simulink library "LIB_TF_G_12_StepControl"  (Simulink 8.6)
settings: Solver=ode45  StartTime=0.0  StopTime=10.0  RelTol=1e-3
PreLoadFcn:
  | if exist('tl_preloadfcn','file'), tl_preloadfcn(gcs,402); end
PostLoadFcn:
  | if exist('tl_postloadfcn','file'), tl_postloadfcn(gcs,402); end
undefined symbols (not defined in the file): ddv, u2, u3
libraries: tllib x4, LIB_TF_G_12_StepControl x1
(part 4 of 7)

== system LIB_TF_G_12_StepControl/TF_G_12_ControlStepExecution/New Step started/Adapt Step Target Value/Temperature Weighted ==
  s8_StepOrderValue : Inport
  u16_Temperature : Inport  Port=2
  e_TemperatureCompensationType : Inport  Port=3
  Action Port : ActionPort
  Data Type Conversion : DataTypeConversion
  If : If  NumInputs=2  IfExpression=u1  ElseIfExpressions=u2
  Merge : Merge  Inputs=3  InitialOutput=64  mask(TL_Merge){data={'date',735951.66799226857}}
      settings: CopyFcn=if exist('tl_reset_reviewflag','file')==2,tl_reset_reviewflag(gcbh);end  DeleteFcn=if exist('delete_tlblock','file')==2,delete_tlblock(gcbh);end  NameChangeFcn=if exist('rename_tlblock','file')==2,rename_tlblock(gcbh);end  OpenFcn=if exist('tl_open_blockdlg','file')==2,tl_open_blockdlg(gcbh);else,open_system(gcbh,'parameter');end
      mask Help: eval(['if exist(''tl_online_help'',''file'') == 2, tl_online_help(''Topic'',''TL_Merge''),else, web([''jar:file:///'',matlabroot,''/help/toolbox/simulink/help.jar!/slref/' lower(get_param(gcbh,'Blocktype')) '.html''], ''-helpbrowser''),end'])
      mask Display: plot([-0.05, 1.05, NaN, -0.05, 1.05],[.01, .01, NaN, .99, .99])
  Relational Operator1 : RelationalOperator  Operator===  OutDataTypeStr=boolean  mask(TL_RelationalOperator){data={'date',735951.66799189814}}
      settings: DeleteFcn=if exist('delete_tlblock','file')==2,delete_tlblock(gcbh);end  NameChangeFcn=if exist('rename_tlblock','file')==2,rename_tlblock(gcbh);end  OpenFcn=if exist('tl_open_blockdlg','file')==2,tl_open_blockdlg(gcbh);else,open_system(gcbh,'parameter');end
      mask Help: eval(['if exist(''tl_online_help'',''file'') == 2, tl_online_help(''Topic'',''TL_RelationalOperator''),else, web([''jar:file:///'',matlabroot,''/help/toolbox/simulink/help.jar!/slref/' lower(get_param(gcbh,'Blocktype')) '.html''], ''-helpbrowser''),end'])
      mask Display: plot([-0.05, 1.05, NaN, -0.05, 1.05],[.01, .01, NaN, .99, .99])
  Relational Operator2 : RelationalOperator  Operator=>  OutDataTypeStr=boolean  mask(TL_RelationalOperator){data={'date',735951.66799165506}}
      settings: DeleteFcn=if exist('delete_tlblock','file')==2,delete_tlblock(gcbh);end  NameChangeFcn=if exist('rename_tlblock','file')==2,rename_tlblock(gcbh);end  OpenFcn=if exist('tl_open_blockdlg','file')==2,tl_open_blockdlg(gcbh);else,open_system(gcbh,'parameter');end
      mask Help: eval(['if exist(''tl_online_help'',''file'') == 2, tl_online_help(''Topic'',''TL_RelationalOperator''),else, web([''jar:file:///'',matlabroot,''/help/toolbox/simulink/help.jar!/slref/' lower(get_param(gcbh,'Blocktype')) '.html''], ''-helpbrowser''),end'])
      mask Display: plot([-0.05, 1.05, NaN, -0.05, 1.05],[.01, .01, NaN, .99, .99])
  Step Order Negative : Subsystem  TreatAsAtomicUnit=on
  Step Order Positive : Subsystem  TreatAsAtomicUnit=on
  Step Order equal 0 : Subsystem  TreatAsAtomicUnit=on
  Zero : Constant  Value=ddv('Common/KS8_ZERO')  mask(TL_Constant){data={'output',{'variable','Common/KS8_ZERO'},'date',735951.66798423615}}
      settings: CopyFcn=if exist('tl_reset_reviewflag','file')==2,tl_reset_reviewflag(gcbh);end  DeleteFcn=if exist('delete_tlblock','file')==2,delete_tlblock(gcbh);end  NameChangeFcn=if exist('rename_tlblock','file')==2,rename_tlblock(gcbh);end  OpenFcn=if exist('tl_open_blockdlg','file')==2,tl_open_blockdlg(gcbh);else,open_system(gcbh,'parameter');end
      mask Help: eval(['if exist(''tl_online_help'',''file'') == 2, tl_online_help(''Topic'',''TL_Constant''),else, web([''jar:file:///'',matlabroot,''/help/toolbox/simulink/help.jar!/slref/' lower(get_param(gcbh,'Blocktype')) '.html''], ''-helpbrowser''),end'])
      mask Display: plot([-0.05, 1.05, NaN, -0.05, 1.05],[.01, .01, NaN, .99, .99])
  Out1 : Outport  InitialOutput=64
  wires:
  s8_StepOrderValue/1 -> Relational Operator1/2, Relational Operator2/2
  Zero/1 -> Relational Operator1/1, Relational Operator2/1
  If/1 -> Step Order equal 0/Action
  Relational Operator1/1 -> If/1
  Relational Operator2/1 -> If/2
  If/2 -> Step Order Negative/Action
  If/3 -> Step Order Positive/Action
  u16_Temperature/1 -> Step Order Positive/1(u16_Temperature), Step Order Negative/1(u16_Temperature)
  e_TemperatureCompensationType/1 -> Step Order Positive/2(e_TemperatureCompensationType)
  Step Order equal 0/1(Out1) -> Merge/1
  Step Order Negative/1(Out1) -> Merge/2
  Step Order Positive/1(Out1) -> Merge/3
  Merge/1 -> Data Type Conversion/1
  Data Type Conversion/1 -> Out1/1

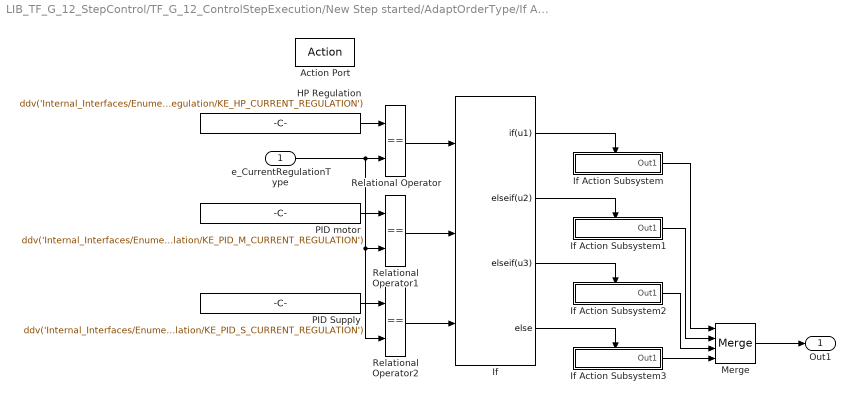
== system LIB_TF_G_12_StepControl/TF_G_12_ControlStepExecution/New Step started/AdaptOrderType/If Action Subsystem ==
  e_CurrentRegulationType : Inport  RequirementInfo={} %GIDa_189e736f_cca1_461e_9619_1829fc2b845e
  Action Port : ActionPort  RequirementInfo={} %GIDa_9c1052a9_2410_4f18_8ef4_d58b860af1af
  HP Regulation : Constant  Value=ddv('Internal_Interfaces/Enumerated_values/Current_Regulation/KE_HP_CURRENT_REGULATION')  mask(TL_Constant){data={'output',{'variable','Internal_Interfaces/Enumerated_values/Current_Regulation/KE_HP_CURRENT_REGULATION'},'date',735951.66798386571}}
      settings: CopyFcn=if exist('tl_reset_reviewflag','file')==2,tl_reset_reviewflag(gcbh);end  DeleteFcn=if exist('delete_tlblock','file')==2,delete_tlblock(gcbh);end  NameChangeFcn=if exist('rename_tlblock','file')==2,rename_tlblock(gcbh);end  OpenFcn=if exist('tl_open_blockdlg','file')==2,tl_open_blockdlg(gcbh);else,open_system(gcbh,'parameter');end
      mask Help: eval(['if exist(''tl_online_help'',''file'') == 2, tl_online_help(''Topic'',''TL_Constant''),else, web([''jar:file:///'',matlabroot,''/help/toolbox/simulink/help.jar!/slref/' lower(get_param(gcbh,'Blocktype')) '.html''], ''-helpbrowser''),end'])
      mask Display: plot([-0.05, 1.05, NaN, -0.05, 1.05],[.01, .01, NaN, .99, .99])
  If : If  RequirementInfo={} %GIDa_8698efec_5c77_4842_b73b_0b3a19be4617  NumInputs=3  IfExpression=u1  ElseIfExpressions=u2,u3
  If Action Subsystem : Subsystem  RequirementInfo={} %GIDa_4ad190b8_12b8_4004_92fb_b3b0c27a36d8  TreatAsAtomicUnit=on
  If Action Subsystem1 : Subsystem  RequirementInfo={} %GIDa_60d8e542_8624_44e2_88e0_16765795048d  TreatAsAtomicUnit=on
  If Action Subsystem2 : Subsystem  RequirementInfo={} %GIDa_c7e553bf_bc73_4930_9906_7d39347ac718  TreatAsAtomicUnit=on
  If Action Subsystem3 : Subsystem  RequirementInfo={} %GIDa_f2cbc51b_f895_475d_9a25_d84b280220b8  TreatAsAtomicUnit=on
  Merge : Merge  RequirementInfo={} %GIDa_b496a0a7_f35d_4795_a756_d7e1fdb3ad5a  Inputs=4  mask(TL_Merge){data={'date',735951.66797821759}}
      settings: CopyFcn=if exist('tl_reset_reviewflag','file')==2,tl_reset_reviewflag(gcbh);end  DeleteFcn=if exist('delete_tlblock','file')==2,delete_tlblock(gcbh);end  NameChangeFcn=if exist('rename_tlblock','file')==2,rename_tlblock(gcbh);end  OpenFcn=if exist('tl_open_blockdlg','file')==2,tl_open_blockdlg(gcbh);else,open_system(gcbh,'parameter');end
      mask Help: eval(['if exist(''tl_online_help'',''file'') == 2, tl_online_help(''Topic'',''TL_Merge''),else, web([''jar:file:///'',matlabroot,''/help/toolbox/simulink/help.jar!/slref/' lower(get_param(gcbh,'Blocktype')) '.html''], ''-helpbrowser''),end'])
      mask Display: plot([-0.05, 1.05, NaN, -0.05, 1.05],[.01, .01, NaN, .99, .99])
  PID Supply : Constant  Value=ddv('Internal_Interfaces/Enumerated_values/Current_Regulation/KE_PID_S_CURRENT_REGULATION')  mask(TL_Constant){data={'output',{'variable','Internal_Interfaces/Enumerated_values/Current_Regulation/KE_PID_S_CURRENT_REGULATION'},'date',735951.66797784728}}
      settings: CopyFcn=if exist('tl_reset_reviewflag','file')==2,tl_reset_reviewflag(gcbh);end  DeleteFcn=if exist('delete_tlblock','file')==2,delete_tlblock(gcbh);end  NameChangeFcn=if exist('rename_tlblock','file')==2,rename_tlblock(gcbh);end  OpenFcn=if exist('tl_open_blockdlg','file')==2,tl_open_blockdlg(gcbh);else,open_system(gcbh,'parameter');end
      mask Help: eval(['if exist(''tl_online_help'',''file'') == 2, tl_online_help(''Topic'',''TL_Constant''),else, web([''jar:file:///'',matlabroot,''/help/toolbox/simulink/help.jar!/slref/' lower(get_param(gcbh,'Blocktype')) '.html''], ''-helpbrowser''),end'])
      mask Display: plot([-0.05, 1.05, NaN, -0.05, 1.05],[.01, .01, NaN, .99, .99])
  PID motor : Constant  Value=ddv('Internal_Interfaces/Enumerated_values/Current_Regulation/KE_PID_M_CURRENT_REGULATION')  mask(TL_Constant){data={'output',{'variable','Internal_Interfaces/Enumerated_values/Current_Regulation/KE_PID_M_CURRENT_REGULATION'},'date',735951.66797747684}}
      settings: CopyFcn=if exist('tl_reset_reviewflag','file')==2,tl_reset_reviewflag(gcbh);end  DeleteFcn=if exist('delete_tlblock','file')==2,delete_tlblock(gcbh);end  NameChangeFcn=if exist('rename_tlblock','file')==2,rename_tlblock(gcbh);end  OpenFcn=if exist('tl_open_blockdlg','file')==2,tl_open_blockdlg(gcbh);else,open_system(gcbh,'parameter');end
      mask Help: eval(['if exist(''tl_online_help'',''file'') == 2, tl_online_help(''Topic'',''TL_Constant''),else, web([''jar:file:///'',matlabroot,''/help/toolbox/simulink/help.jar!/slref/' lower(get_param(gcbh,'Blocktype')) '.html''], ''-helpbrowser''),end'])
      mask Display: plot([-0.05, 1.05, NaN, -0.05, 1.05],[.01, .01, NaN, .99, .99])
  Relational Operator : RelationalOperator  Operator===  OutDataTypeStr=boolean  mask(TL_RelationalOperator){data={'date',735951.66797711805}}
      settings: DeleteFcn=if exist('delete_tlblock','file')==2,delete_tlblock(gcbh);end  NameChangeFcn=if exist('rename_tlblock','file')==2,rename_tlblock(gcbh);end  OpenFcn=if exist('tl_open_blockdlg','file')==2,tl_open_blockdlg(gcbh);else,open_system(gcbh,'parameter');end
      mask Help: eval(['if exist(''tl_online_help'',''file'') == 2, tl_online_help(''Topic'',''TL_RelationalOperator''),else, web([''jar:file:///'',matlabroot,''/help/toolbox/simulink/help.jar!/slref/' lower(get_param(gcbh,'Blocktype')) '.html''], ''-helpbrowser''),end'])
      mask Display: plot([-0.05, 1.05, NaN, -0.05, 1.05],[.01, .01, NaN, .99, .99])
  Relational Operator1 : RelationalOperator  Operator===  OutDataTypeStr=boolean  mask(TL_RelationalOperator){data={'date',735951.66797687497}}
      settings: DeleteFcn=if exist('delete_tlblock','file')==2,delete_tlblock(gcbh);end  NameChangeFcn=if exist('rename_tlblock','file')==2,rename_tlblock(gcbh);end  OpenFcn=if exist('tl_open_blockdlg','file')==2,tl_open_blockdlg(gcbh);else,open_system(gcbh,'parameter');end
      mask Help: eval(['if exist(''tl_online_help'',''file'') == 2, tl_online_help(''Topic'',''TL_RelationalOperator''),else, web([''jar:file:///'',matlabroot,''/help/toolbox/simulink/help.jar!/slref/' lower(get_param(gcbh,'Blocktype')) '.html''], ''-helpbrowser''),end'])
      mask Display: plot([-0.05, 1.05, NaN, -0.05, 1.05],[.01, .01, NaN, .99, .99])
  Relational Operator2 : RelationalOperator  Operator===  OutDataTypeStr=boolean  mask(TL_RelationalOperator){data={'date',735951.66797660885}}
      settings: DeleteFcn=if exist('delete_tlblock','file')==2,delete_tlblock(gcbh);end  NameChangeFcn=if exist('rename_tlblock','file')==2,rename_tlblock(gcbh);end  OpenFcn=if exist('tl_open_blockdlg','file')==2,tl_open_blockdlg(gcbh);else,open_system(gcbh,'parameter');end
      mask Help: eval(['if exist(''tl_online_help'',''file'') == 2, tl_online_help(''Topic'',''TL_RelationalOperator''),else, web([''jar:file:///'',matlabroot,''/help/toolbox/simulink/help.jar!/slref/' lower(get_param(gcbh,'Blocktype')) '.html''], ''-helpbrowser''),end'])
      mask Display: plot([-0.05, 1.05, NaN, -0.05, 1.05],[.01, .01, NaN, .99, .99])
  Out1 : Outport  RequirementInfo={} %GIDa_50a863bf_4662_4db8_95fd_37f32455ccc3
  wires:
  If/1 -> If Action Subsystem/Action
  If/2 -> If Action Subsystem1/Action
  If/3 -> If Action Subsystem2/Action
  If/4 -> If Action Subsystem3/Action
  If Action Subsystem/1(Out1) -> Merge/1
  If Action Subsystem1/1(Out1) -> Merge/2
  If Action Subsystem2/1(Out1) -> Merge/3
  If Action Subsystem3/1(Out1) -> Merge/4
  Merge/1 -> Out1/1
  HP Regulation/1 -> Relational Operator/1
  e_CurrentRegulationType/1 -> Relational Operator/2, Relational Operator1/2, Relational Operator2/2
  Relational Operator/1 -> If/1
  Relational Operator1/1 -> If/2
  Relational Operator2/1 -> If/3
  PID motor/1 -> Relational Operator1/1
  PID Supply/1 -> Relational Operator2/1

== system LIB_TF_G_12_StepControl/TF_G_12_ControlStepExecution/New Step started/AdaptOrderType/If Action Subsystem1 ==
  Action Port : ActionPort  RequirementInfo={} %GIDa_8c90ece7_90af_483e_9cad_cdc68c903bb6
  KU8_NO_STEP_TYPE : Constant  RequirementInfo={} %GIDa_88d5ae82_7c73_413a_a46d_5c66edb192c1  Value=ddv('BFE/Step_Def/KU8_NO_STEP_TYPE')  OutDataTypeStr=uint8  mask(TL_Constant){data={'output',{'variable','BFE/Step_Def/KU8_NO_STEP_TYPE'},'date',735951.66797635413}}
      settings: CopyFcn=if exist('tl_reset_reviewflag','file')==2,tl_reset_reviewflag(gcbh);end  DeleteFcn=if exist('delete_tlblock','file')==2,delete_tlblock(gcbh);end  NameChangeFcn=if exist('rename_tlblock','file')==2,rename_tlblock(gcbh);end  OpenFcn=if exist('tl_open_blockdlg','file')==2,tl_open_blockdlg(gcbh);else,open_system(gcbh,'parameter');end
      mask Help: eval(['if exist(''tl_online_help'',''file'') == 2, tl_online_help(''Topic'',''TL_Constant''),else, web([''jar:file:///'',matlabroot,''/help/toolbox/simulink/help.jar!/slref/' lower(get_param(gcbh,'Blocktype')) '.html''], ''-helpbrowser''),end'])
      mask Display: plot([-0.05, 1.05, NaN, -0.05, 1.05],[.01, .01, NaN, .99, .99])
  Out1 : Outport  RequirementInfo={} %GIDa_4ff01bec_1f37_45e3_ae87_576e41db2508  InitialOutput=7
  wires:
  KU8_NO_STEP_TYPE/1 -> Out1/1

== system LIB_TF_G_12_StepControl/TF_G_12_ControlStepExecution/New Step started/AdaptOrderType/If Action Subsystem2 ==
  u8OrderType : Inport  RequirementInfo={} %GIDa_12107d9c_51c6_4b9c_ba46_1c9b53391efd
  Action Port : ActionPort  RequirementInfo={} %GIDa_1aa301e4_226a_435e_a06b_635fcf600117
  Out1 : Outport  RequirementInfo={} %GIDa_f21eaf6f_27b3_4c29_92cc_8d5822c08ad3  InitialOutput=7
  wires:
  u8OrderType/1 -> Out1/1

== system LIB_TF_G_12_StepControl/TF_G_12_ControlStepExecution/New Step started/Ramp step characteristics computation/If Action Subsystem ==
  In1 : Inport
  Action Port : ActionPort
  Gain : Gain  Gain=128  OutDataTypeStr=int32  mask(TL_Gain){data={'output',{'type','Int32'},'gain',{'variable','BFE/KU16_HIGH_RESC_PWM'},'date',735951.6679730555}}
      settings: CopyFcn=if exist('tl_reset_reviewflag','file')==2,tl_reset_reviewflag(gcbh);end  DeleteFcn=if exist('delete_tlblock','file')==2,delete_tlblock(gcbh);end  NameChangeFcn=if exist('rename_tlblock','file')==2,rename_tlblock(gcbh);end  OpenFcn=if exist('tl_open_blockdlg','file')==2,tl_open_blockdlg(gcbh);else,open_system(gcbh,'parameter');end
      mask Help: eval(['if exist(''tl_online_help'',''file'') == 2, tl_online_help(''Topic'',''TL_Gain''),else, web([''jar:file:///'',matlabroot,''/help/toolbox/simulink/help.jar!/slref/' lower(get_param(gcbh,'Blocktype')) '.html''], ''-helpbrowser''),end'])
      mask Display: plot([0, .9, 0],[.05, .5, .95])
  Out1 : Outport  InitialOutput=0
  wires:
  In1/1 -> Gain/1
  Gain/1 -> Out1/1

== system LIB_TF_G_12_StepControl/TF_G_12_ControlStepExecution/New Step started/Ramp step characteristics computation/If Action Subsystem1 ==
  note: 1 lsb = 1mA
  note: 8192 lsb = 500 mA
  In1 : Inport
  Action Port : ActionPort
  Constant : Constant  Value=500  OutDataTypeStr=int32  mask(TL_Constant){data={'date',735951.66797256947}}
      settings: CopyFcn=if exist('tl_reset_reviewflag','file')==2,tl_reset_reviewflag(gcbh);end  DeleteFcn=if exist('delete_tlblock','file')==2,delete_tlblock(gcbh);end  NameChangeFcn=if exist('rename_tlblock','file')==2,rename_tlblock(gcbh);end  OpenFcn=if exist('tl_open_blockdlg','file')==2,tl_open_blockdlg(gcbh);else,open_system(gcbh,'parameter');end
      mask Help: eval(['if exist(''tl_online_help'',''file'') == 2, tl_online_help(''Topic'',''TL_Constant''),else, web([''jar:file:///'',matlabroot,''/help/toolbox/simulink/help.jar!/slref/' lower(get_param(gcbh,'Blocktype')) '.html''], ''-helpbrowser''),end'])
      mask Display: plot([-0.05, 1.05, NaN, -0.05, 1.05],[.01, .01, NaN, .99, .99])
  Constant1 : Constant  Value=ddv('BFE/KU16_HIGH_RESC_NOM_CURRENT')  mask(TL_Constant){data={'output',{'variable','BFE/KU16_HIGH_RESC_NOM_CURRENT'},'date',735951.66797219904}}
      settings: CopyFcn=if exist('tl_reset_reviewflag','file')==2,tl_reset_reviewflag(gcbh);end  DeleteFcn=if exist('delete_tlblock','file')==2,delete_tlblock(gcbh);end  NameChangeFcn=if exist('rename_tlblock','file')==2,rename_tlblock(gcbh);end  OpenFcn=if exist('tl_open_blockdlg','file')==2,tl_open_blockdlg(gcbh);else,open_system(gcbh,'parameter');end
      mask Help: eval(['if exist(''tl_online_help'',''file'') == 2, tl_online_help(''Topic'',''TL_Constant''),else, web([''jar:file:///'',matlabroot,''/help/toolbox/simulink/help.jar!/slref/' lower(get_param(gcbh,'Blocktype')) '.html''], ''-helpbrowser''),end'])
      mask Display: plot([-0.05, 1.05, NaN, -0.05, 1.05],[.01, .01, NaN, .99, .99])
  Product : Product  Inputs=*/  OutDataTypeStr=int32  RndMeth=Zero  mask(TL_Product){data={'output',{'type','Int32'},'exceptionhandling',0,'autoscaling',{'mode',2},'date',735951.66797180555}}
      settings: CopyFcn=if exist('tl_reset_reviewflag','file')==2,tl_reset_reviewflag(gcbh);end  DeleteFcn=if exist('delete_tlblock','file')==2,delete_tlblock(gcbh);end  NameChangeFcn=if exist('rename_tlblock','file')==2,rename_tlblock(gcbh);end  OpenFcn=if exist('tl_open_blockdlg','file')==2,tl_open_blockdlg(gcbh);else,open_system(gcbh,'parameter');end
      mask Help: eval(['if exist(''tl_online_help'',''file'') == 2, tl_online_help(''Topic'',''TL_Product''),else, web([''jar:file:///'',matlabroot,''/help/toolbox/simulink/help.jar!/slref/' lower(get_param(gcbh,'Blocktype')) '.html''], ''-helpbrowser''),end'])
      mask Display: plot([-0.05, 1.05, NaN, -0.05, 1.05],[.01, .01, NaN, .99, .99])
  Product1 : Product  Inputs=**  RndMeth=Zero  mask(TL_Product){data={'output',{'name','u32LocRscMotorCurrent','type','Int32'},'exceptionhandling',0,'date',735951.66797142359}}
      settings: CopyFcn=if exist('tl_reset_reviewflag','file')==2,tl_reset_reviewflag(gcbh);end  DeleteFcn=if exist('delete_tlblock','file')==2,delete_tlblock(gcbh);end  NameChangeFcn=if exist('rename_tlblock','file')==2,rename_tlblock(gcbh);end  OpenFcn=if exist('tl_open_blockdlg','file')==2,tl_open_blockdlg(gcbh);else,open_system(gcbh,'parameter');end
      mask Help: eval(['if exist(''tl_online_help'',''file'') == 2, tl_online_help(''Topic'',''TL_Product''),else, web([''jar:file:///'',matlabroot,''/help/toolbox/simulink/help.jar!/slref/' lower(get_param(gcbh,'Blocktype')) '.html''], ''-helpbrowser''),end'])
      mask Display: plot([-0.05, 1.05, NaN, -0.05, 1.05],[.01, .01, NaN, .99, .99])
  Out1 : Outport  InitialOutput=0
  wires:
  In1/1 -> Product1/2
  Product1/1 -> Product/1
  Product/1 -> Out1/1
  Constant/1 -> Product/2
  Constant1/1 -> Product1/1

== system LIB_TF_G_12_StepControl/TF_G_12_ControlStepExecution/New Step started/Ramp step characteristics computation/If Action Subsystem2 ==
  In1 : Inport
  In2 : Inport  Port=2
  Action Port : ActionPort
  Constant : Constant  Value=250  mask(TL_Constant){data={'output',{'variable','BFE/KUS_MOTOR_VOLTAGE_ORDER_RES'},'date',735951.66797107644}}
      settings: CopyFcn=if exist('tl_reset_reviewflag','file')==2,tl_reset_reviewflag(gcbh);end  DeleteFcn=if exist('delete_tlblock','file')==2,delete_tlblock(gcbh);end  NameChangeFcn=if exist('rename_tlblock','file')==2,rename_tlblock(gcbh);end  OpenFcn=if exist('tl_open_blockdlg','file')==2,tl_open_blockdlg(gcbh);else,open_system(gcbh,'parameter');end
      mask Help: eval(['if exist(''tl_online_help'',''file'') == 2, tl_online_help(''Topic'',''TL_Constant''),else, web([''jar:file:///'',matlabroot,''/help/toolbox/simulink/help.jar!/slref/' lower(get_param(gcbh,'Blocktype')) '.html''], ''-helpbrowser''),end'])
      mask Display: plot([-0.05, 1.05, NaN, -0.05, 1.05],[.01, .01, NaN, .99, .99])
  Constant1 : Constant  Value=100  mask(TL_Constant){data={'output',{'variable','BFE/KU16_HIGH_RESC_DEN_VOLT'},'date',735951.66797070601}}
      settings: CopyFcn=if exist('tl_reset_reviewflag','file')==2,tl_reset_reviewflag(gcbh);end  DeleteFcn=if exist('delete_tlblock','file')==2,delete_tlblock(gcbh);end  NameChangeFcn=if exist('rename_tlblock','file')==2,rename_tlblock(gcbh);end  OpenFcn=if exist('tl_open_blockdlg','file')==2,tl_open_blockdlg(gcbh);else,open_system(gcbh,'parameter');end
      mask Help: eval(['if exist(''tl_online_help'',''file'') == 2, tl_online_help(''Topic'',''TL_Constant''),else, web([''jar:file:///'',matlabroot,''/help/toolbox/simulink/help.jar!/slref/' lower(get_param(gcbh,'Blocktype')) '.html''], ''-helpbrowser''),end'])
      mask Display: plot([-0.05, 1.05, NaN, -0.05, 1.05],[.01, .01, NaN, .99, .99])
  Gain : Gain  Gain=128  ParamDataTypeStr=int32  OutDataTypeStr=int32  mask(TL_Gain){data={'output',{'type','Int32'},'gain',{'variable','BFE/KU16_HIGH_RESC_NOM_VOLT'},'date',735951.66797028936}}
      settings: CopyFcn=if exist('tl_reset_reviewflag','file')==2,tl_reset_reviewflag(gcbh);end  DeleteFcn=if exist('delete_tlblock','file')==2,delete_tlblock(gcbh);end  NameChangeFcn=if exist('rename_tlblock','file')==2,rename_tlblock(gcbh);end  OpenFcn=if exist('tl_open_blockdlg','file')==2,tl_open_blockdlg(gcbh);else,open_system(gcbh,'parameter');end
      mask Help: eval(['if exist(''tl_online_help'',''file'') == 2, tl_online_help(''Topic'',''TL_Gain''),else, web([''jar:file:///'',matlabroot,''/help/toolbox/simulink/help.jar!/slref/' lower(get_param(gcbh,'Blocktype')) '.html''], ''-helpbrowser''),end'])
      mask Display: plot([0, .9, 0],[.05, .5, .95])
  Product : Product  Inputs=*/  OutDataTypeStr=int32  RndMeth=Zero  mask(TL_Product){data={'output',{'type','UInt16'},'date',735951.66796975699}}
      settings: CopyFcn=if exist('tl_reset_reviewflag','file')==2,tl_reset_reviewflag(gcbh);end  DeleteFcn=if exist('delete_tlblock','file')==2,delete_tlblock(gcbh);end  NameChangeFcn=if exist('rename_tlblock','file')==2,rename_tlblock(gcbh);end  OpenFcn=if exist('tl_open_blockdlg','file')==2,tl_open_blockdlg(gcbh);else,open_system(gcbh,'parameter');end
      mask Help: eval(['if exist(''tl_online_help'',''file'') == 2, tl_online_help(''Topic'',''TL_Product''),else, web([''jar:file:///'',matlabroot,''/help/toolbox/simulink/help.jar!/slref/' lower(get_param(gcbh,'Blocktype')) '.html''], ''-helpbrowser''),end'])
      mask Display: plot([-0.05, 1.05, NaN, -0.05, 1.05],[.01, .01, NaN, .99, .99])
  Product1 : Product  Inputs=**  OutDataTypeStr=int32  RndMeth=Zero  mask(TL_Product){data={'output',{'type','Int32'},'date',735951.6679693982}}
      settings: CopyFcn=if exist('tl_reset_reviewflag','file')==2,tl_reset_reviewflag(gcbh);end  DeleteFcn=if exist('delete_tlblock','file')==2,delete_tlblock(gcbh);end  NameChangeFcn=if exist('rename_tlblock','file')==2,rename_tlblock(gcbh);end  OpenFcn=if exist('tl_open_blockdlg','file')==2,tl_open_blockdlg(gcbh);else,open_system(gcbh,'parameter');end
      mask Help: eval(['if exist(''tl_online_help'',''file'') == 2, tl_online_help(''Topic'',''TL_Product''),else, web([''jar:file:///'',matlabroot,''/help/toolbox/simulink/help.jar!/slref/' lower(get_param(gcbh,'Blocktype')) '.html''], ''-helpbrowser''),end'])
      mask Display: plot([-0.05, 1.05, NaN, -0.05, 1.05],[.01, .01, NaN, .99, .99])
  Product2 : Product  Inputs=*/  OutDataTypeStr=int32  RndMeth=Zero  mask(TL_Product){data={'output',{'type','Int32'},'exceptionhandling',0,'date',735951.66796903941}}
      settings: CopyFcn=if exist('tl_reset_reviewflag','file')==2,tl_reset_reviewflag(gcbh);end  DeleteFcn=if exist('delete_tlblock','file')==2,delete_tlblock(gcbh);end  NameChangeFcn=if exist('rename_tlblock','file')==2,rename_tlblock(gcbh);end  OpenFcn=if exist('tl_open_blockdlg','file')==2,tl_open_blockdlg(gcbh);else,open_system(gcbh,'parameter');end
      mask Help: eval(['if exist(''tl_online_help'',''file'') == 2, tl_online_help(''Topic'',''TL_Product''),else, web([''jar:file:///'',matlabroot,''/help/toolbox/simulink/help.jar!/slref/' lower(get_param(gcbh,'Blocktype')) '.html''], ''-helpbrowser''),end'])
      mask Display: plot([-0.05, 1.05, NaN, -0.05, 1.05],[.01, .01, NaN, .99, .99])
  Out1 : Outport  InitialOutput=0
  wires:
  In2/1 -> Product/1
  Constant/1 -> Product/2
  In1/1 -> Gain/1
  Product/1 -> Product1/2
  Gain/1 -> Product1/1
  Product1/1 -> Product2/1
  Product2/1 -> Out1/1
  Constant1/1 -> Product2/2

== system LIB_TF_G_12_StepControl/TF_G_12_ManageEndingStep/Step execution in progress/ManageAdaptiveCurrentInterruptionPoint (Comfort Belt Functions)/Current Int Point Opt Activated ==
  u8AdaptiveCurrentLimitation : Inport  RequirementInfo={} %GIDa_d520d43c_8b3b_4f1a_b65f_f5e1acb92388
  u32MotorCurrent : Inport  RequirementInfo={} %GIDa_eebca9ca_2751_4dea_9a4f_f23b39810d46  Port=2
  u16Temperature : Inport  RequirementInfo={} %GIDa_8991d2a0_20b4_4be7_9e1d_2669c6999acc  Port=3
  Action Port : ActionPort  RequirementInfo={} %GIDa_8f315547_3222_4786_8102_193294aef773
  Constant : Constant  RequirementInfo={} %GIDa_404df9ca_9c91_4b4d_aea1_b6852152ed24  Value=ddv('Common/KU8_ZERO')  OutDataTypeStr=uint8  SampleTime=-1  mask(TL_Constant){data={'output',{'variable','Common/KU8_ZERO'},'date',735951.66848394671}}
      settings: CopyFcn=if exist('tl_reset_reviewflag','file')==2,tl_reset_reviewflag(gcbh);end  DeleteFcn=if exist('delete_tlblock','file')==2,delete_tlblock(gcbh);end  NameChangeFcn=if exist('rename_tlblock','file')==2,rename_tlblock(gcbh);end  OpenFcn=if exist('tl_open_blockdlg','file')==2,tl_open_blockdlg(gcbh);else,open_system(gcbh,'parameter');end
      mask Help: eval(['if exist(''tl_online_help'',''file'') == 2, tl_online_help(''Topic'',''TL_Constant''),else, web([''jar:file:///'',matlabroot,''/help/toolbox/simulink/help.jar!/slref/' lower(get_param(gcbh,'Blocktype')) '.html''], ''-helpbrowser''),end'])
      mask Display: plot([-0.05, 1.05, NaN, -0.05, 1.05],[.01, .01, NaN, .99, .99])
  Constant1 : Constant  RequirementInfo={} %GIDa_5533d7b1_0bbd_4c47_89d8_547f66f9a94f  Value=ddv('BFE_Config_Data/CFG_KAU16_ADAPTATIVE_CURRENT_LIMIT')  OutDataTypeStr=uint16  SampleTime=-1  mask(TL_Constant){data={'output',{'variable','BFE_Config_Data/CFG_KAU16_ADAPTATIVE_CURRENT_LIMIT'},'date',735951.66848356486}}
      settings: CopyFcn=if exist('tl_reset_reviewflag','file')==2,tl_reset_reviewflag(gcbh);end  DeleteFcn=if exist('delete_tlblock','file')==2,delete_tlblock(gcbh);end  NameChangeFcn=if exist('rename_tlblock','file')==2,rename_tlblock(gcbh);end  OpenFcn=if exist('tl_open_blockdlg','file')==2,tl_open_blockdlg(gcbh);else,open_system(gcbh,'parameter');end
      mask Help: eval(['if exist(''tl_online_help'',''file'') == 2, tl_online_help(''Topic'',''TL_Constant''),else, web([''jar:file:///'',matlabroot,''/help/toolbox/simulink/help.jar!/slref/' lower(get_param(gcbh,'Blocktype')) '.html''], ''-helpbrowser''),end'])
      mask Display: plot([-0.05, 1.05, NaN, -0.05, 1.05],[.01, .01, NaN, .99, .99])
  KB_FALSE : Constant  RequirementInfo={} %GIDa_9edde50e_bd2a_4077_84c3_2221ede5e359  Value=ddv('BFE/KB_FALSE')  OutDataTypeStr=boolean  SampleTime=-1  mask(TL_Constant){data={'output',{'variable','BFE/KB_FALSE'},'date',735951.66848295135}}
      settings: CopyFcn=if exist('tl_reset_reviewflag','file')==2,tl_reset_reviewflag(gcbh);end  DeleteFcn=if exist('delete_tlblock','file')==2,delete_tlblock(gcbh);end  NameChangeFcn=if exist('rename_tlblock','file')==2,rename_tlblock(gcbh);end  OpenFcn=if exist('tl_open_blockdlg','file')==2,tl_open_blockdlg(gcbh);else,open_system(gcbh,'parameter');end
      mask Help: eval(['if exist(''tl_online_help'',''file'') == 2, tl_online_help(''Topic'',''TL_Constant''),else, web([''jar:file:///'',matlabroot,''/help/toolbox/simulink/help.jar!/slref/' lower(get_param(gcbh,'Blocktype')) '.html''], ''-helpbrowser''),end'])
      mask Display: plot([-0.05, 1.05, NaN, -0.05, 1.05],[.01, .01, NaN, .99, .99])
  Product : Product  RequirementInfo={} %GIDa_b5b5b953_fa4b_4b0a_b115_5afdc5fd921b  Inputs=**  RndMeth=Zero  mask(TL_Product){data={'output',{'type','UInt32'},'date',735951.6684825694}}
      settings: CopyFcn=if exist('tl_reset_reviewflag','file')==2,tl_reset_reviewflag(gcbh);end  DeleteFcn=if exist('delete_tlblock','file')==2,delete_tlblock(gcbh);end  NameChangeFcn=if exist('rename_tlblock','file')==2,rename_tlblock(gcbh);end  OpenFcn=if exist('tl_open_blockdlg','file')==2,tl_open_blockdlg(gcbh);else,open_system(gcbh,'parameter');end
      mask Help: eval(['if exist(''tl_online_help'',''file'') == 2, tl_online_help(''Topic'',''TL_Product''),else, web([''jar:file:///'',matlabroot,''/help/toolbox/simulink/help.jar!/slref/' lower(get_param(gcbh,'Blocktype')) '.html''], ''-helpbrowser''),end'])
      mask Display: plot([-0.05, 1.05, NaN, -0.05, 1.05],[.01, .01, NaN, .99, .99])
  Relational Operator : RelationalOperator  RequirementInfo={} %GIDa_28898a34_f038_4852_a694_0730bf70f0c2  Operator===  OutDataTypeStr=boolean  mask(TL_RelationalOperator){data={'date',735951.66848222225}}
      settings: DeleteFcn=if exist('delete_tlblock','file')==2,delete_tlblock(gcbh);end  NameChangeFcn=if exist('rename_tlblock','file')==2,rename_tlblock(gcbh);end  OpenFcn=if exist('tl_open_blockdlg','file')==2,tl_open_blockdlg(gcbh);else,open_system(gcbh,'parameter');end
      mask Help: eval(['if exist(''tl_online_help'',''file'') == 2, tl_online_help(''Topic'',''TL_RelationalOperator''),else, web([''jar:file:///'',matlabroot,''/help/toolbox/simulink/help.jar!/slref/' lower(get_param(gcbh,'Blocktype')) '.html''], ''-helpbrowser''),end'])
      mask Display: plot([-0.05, 1.05, NaN, -0.05, 1.05],[.01, .01, NaN, .99, .99])
  Relational Operator1 : RelationalOperator  RequirementInfo={} %GIDa_32b9055d_f184_4cda_8744_e784013df450  Operator=<=  OutDataTypeStr=boolean  mask(TL_RelationalOperator){data={'date',735951.66848196764}}
      settings: DeleteFcn=if exist('delete_tlblock','file')==2,delete_tlblock(gcbh);end  NameChangeFcn=if exist('rename_tlblock','file')==2,rename_tlblock(gcbh);end  OpenFcn=if exist('tl_open_blockdlg','file')==2,tl_open_blockdlg(gcbh);else,open_system(gcbh,'parameter');end
      mask Help: eval(['if exist(''tl_online_help'',''file'') == 2, tl_online_help(''Topic'',''TL_RelationalOperator''),else, web([''jar:file:///'',matlabroot,''/help/toolbox/simulink/help.jar!/slref/' lower(get_param(gcbh,'Blocktype')) '.html''], ''-helpbrowser''),end'])
      mask Display: plot([-0.05, 1.05, NaN, -0.05, 1.05],[.01, .01, NaN, .99, .99])
  Scope : Scope  NumInputPorts=3
  SelectAdaptativFactor : Lookup_n-D  RequirementInfo={} %GIDa_6d14e83f_aff6_4e91_87e5_115fde0656b4  NumberOfTableDimensions=1  BreakpointsForDimension1=ddv('BFE_Config_Data/CFG_au16AdaptCurrentLimitTempIdx')  BreakpointsForDimension2=[1:3]  IndexSearchMethod=Linear search  Table=ddv('BFE_Config_Data/CFG_au8AdaptCurrentLimitFactors')  ExtrapMethod=Clip  OutDataTypeStr=uint8  InputSameDT=on  mask(TL_Lookup1D){data={'input',{'variable','BFE_Config_Data/CFG_au16AdaptCurrentLimitTempIdx'},'output',{'type','UInt8'},'table',{'variable','BFE_Config_Data/CFG_au8AdaptCurrentLimitFactors'},'date',735951.6684816319}}
      settings: CopyFcn=if exist('tl_reset_reviewflag','file')==2,tl_reset_reviewflag(gcbh);end  DeleteFcn=if exist('delete_tlblock','file')==2,delete_tlblock(gcbh);end  NameChangeFcn=if exist('rename_tlblock','file')==2,rename_tlblock(gcbh);end  OpenFcn=if exist('tl_open_blockdlg','file')==2,tl_open_blockdlg(gcbh);else,open_system(gcbh,'parameter');end
      mask Help: eval(['if exist(''tl_online_help'',''file'') == 2, tl_online_help(''Topic'',''TL_Lookup1D''),else, web([''jar:file:///'',matlabroot,''/help/toolbox/simulink/help.jar!/slref/' lower(get_param(gcbh,'Blocktype')) '.html''], ''-helpbrowser''),end'])
      mask Display: plot([-0.05, 1.05, NaN, -0.05, 1.05],[.01, .01, NaN, .99, .99])
  Selector : Selector  RequirementInfo={} %GIDa_9221b351_9e2b_4e66_9397_086f9bb8ceb5  IndexMode=Zero-based  IndexOptions=Index vector (port)  Indices=[1 3]  OutputSizes=1
  Switch : Switch  RequirementInfo={} %GIDa_52caf6ac_91f4_4c36_b614_caea4b5168aa  Criteria=u2 ~= 0  mask(TL_Switch){data={'output',{'type','Bool'},'date',735951.66848043981}}
      settings: CopyFcn=if exist('tl_reset_reviewflag','file')==2,tl_reset_reviewflag(gcbh);end  DeleteFcn=if exist('delete_tlblock','file')==2,delete_tlblock(gcbh);end  NameChangeFcn=if exist('rename_tlblock','file')==2,rename_tlblock(gcbh);end  OpenFcn=if exist('tl_open_blockdlg','file')==2,tl_open_blockdlg(gcbh);else,open_system(gcbh,'parameter');end
      mask Help: eval(['if exist(''tl_online_help'',''file'') == 2, tl_online_help(''Topic'',''TL_Switch''),else, web([''jar:file:///'',matlabroot,''/help/toolbox/simulink/help.jar!/slref/' lower(get_param(gcbh,'Blocktype')) '.html''], ''-helpbrowser''),end'])
      mask Display: plot([-0.05, 1.05, NaN, -0.05, 1.05],[.01, .01, NaN, .99, .99])
  bInterruptStep : Outport  RequirementInfo={} %GIDa_ec579278_a955_4955_a9f1_7578aaad8586
  wires:
  Constant/1 -> Relational Operator/1
  u8AdaptiveCurrentLimitation/1 -> Relational Operator/2, Selector/2
  Constant1/1 -> Selector/1
  u32MotorCurrent/1 -> Relational Operator1/2
  Selector/1 -> Scope/1, Product/1
  Product/1 -> Scope/2, Relational Operator1/1
  Relational Operator/1 -> Switch/2
  Relational Operator1/1 -> Switch/3
  SelectAdaptativFactor/1 -> Scope/3, Product/2
  u16Temperature/1 -> SelectAdaptativFactor/1
  Switch/1 -> bInterruptStep/1
  KB_FALSE/1 -> Switch/1

== system LIB_TF_G_12_StepControl/TF_G_12_ManageEndingStep/Step execution in progress/ManageAdaptiveCurrentInterruptionPoint (Comfort Belt Functions)/Current Int Point Opt Deactivated ==
  Action Port : ActionPort  RequirementInfo={} %GIDa_a8d211dc_8f02_4d3b_82a3_17f3d4532e6a
  KB_FALSE : Constant  RequirementInfo={} %GIDa_a044f4a2_a069_45d6_84ee_e4155b0aedec  Value=ddv('BFE/KB_FALSE')  OutDataTypeStr=boolean  SampleTime=-1  mask(TL_Constant){data={'output',{'variable','BFE/KB_FALSE'},'date',735951.66847995366}}
      settings: CopyFcn=if exist('tl_reset_reviewflag','file')==2,tl_reset_reviewflag(gcbh);end  DeleteFcn=if exist('delete_tlblock','file')==2,delete_tlblock(gcbh);end  NameChangeFcn=if exist('rename_tlblock','file')==2,rename_tlblock(gcbh);end  OpenFcn=if exist('tl_open_blockdlg','file')==2,tl_open_blockdlg(gcbh);else,open_system(gcbh,'parameter');end
      mask Help: eval(['if exist(''tl_online_help'',''file'') == 2, tl_online_help(''Topic'',''TL_Constant''),else, web([''jar:file:///'',matlabroot,''/help/toolbox/simulink/help.jar!/slref/' lower(get_param(gcbh,'Blocktype')) '.html''], ''-helpbrowser''),end'])
      mask Display: plot([-0.05, 1.05, NaN, -0.05, 1.05],[.01, .01, NaN, .99, .99])
  bInterruptStep : Outport  RequirementInfo={} %GIDa_3dd57ca1_bc24_46ef_9fd1_fdb590407adf  InitialOutput=0
  wires:
  KB_FALSE/1 -> bInterruptStep/1

== system LIB_TF_G_12_StepControl/TF_G_12_ManageEndingStep/Step execution in progress/ManageBeltBlocked (HES sensors)/Belt Blocked Opt Activated ==
  bBeltBlockedControlled : Inport  RequirementInfo={} %GIDa_21b4cb51_41d3_491b_b961_8fd0df082f49
  s32BeltSpeed : Inport  RequirementInfo={} %GIDa_1a45e986_6568_42b9_b4ab_bbb37b644456  Port=2
  Action Port : ActionPort  RequirementInfo={} %GIDa_3f5a3ea4_8ca6_45f8_b9ab_7ed678853d65
  B_TRUE : Constant  RequirementInfo={} %GIDa_4f999615_9828_4dff_a198_6441ae5bad18  Value=ddv('Common/KS32_ZERO')  OutDataTypeStr=int32  SampleTime=-1  mask(TL_Constant){data={'output',{'variable','Common/KS32_ZERO'},'date',735951.66847905098}}
      settings: CopyFcn=if exist('tl_reset_reviewflag','file')==2,tl_reset_reviewflag(gcbh);end  DeleteFcn=if exist('delete_tlblock','file')==2,delete_tlblock(gcbh);end  NameChangeFcn=if exist('rename_tlblock','file')==2,rename_tlblock(gcbh);end  OpenFcn=if exist('tl_open_blockdlg','file')==2,tl_open_blockdlg(gcbh);else,open_system(gcbh,'parameter');end
      mask Help: eval(['if exist(''tl_online_help'',''file'') == 2, tl_online_help(''Topic'',''TL_Constant''),else, web([''jar:file:///'',matlabroot,''/help/toolbox/simulink/help.jar!/slref/' lower(get_param(gcbh,'Blocktype')) '.html''], ''-helpbrowser''),end'])
      mask Display: plot([-0.05, 1.05, NaN, -0.05, 1.05],[.01, .01, NaN, .99, .99])
  ManageBeltBlocked : Logic  RequirementInfo={} %GIDa_8fd3ce33_5d76_49a7_bdad_5b79dc26edad  AllPortsSameDT=off  OutDataTypeStr=boolean  mask(TL_LogicalOperator){data={'date',735951.66847868054}}
      settings: DeleteFcn=if exist('delete_tlblock','file')==2,delete_tlblock(gcbh);end  NameChangeFcn=if exist('rename_tlblock','file')==2,rename_tlblock(gcbh);end  OpenFcn=if exist('tl_open_blockdlg','file')==2,tl_open_blockdlg(gcbh);else,open_system(gcbh,'parameter');end
      mask Help: eval(['if exist(''tl_online_help'',''file'') == 2, tl_online_help(''Topic'',''TL_LogicalOperator''),else, web([''jar:file:///'',matlabroot,''/help/toolbox/simulink/help.jar!/slref/' lower(get_param(gcbh,'Blocktype')) '.html''], ''-helpbrowser''),end'])
      mask Display: plot([-0.05, 1.05, NaN, -0.05, 1.05],[.01, .01, NaN, .99, .99])
  RelationalOperator_bAccelerationLow : RelationalOperator  RequirementInfo={} %GIDa_1bbef016_f965_4fae_8632_c9f001a16ad3  Operator===  OutDataTypeStr=boolean  mask(TL_RelationalOperator){data={'date',735951.66847842594}}
      settings: DeleteFcn=if exist('delete_tlblock','file')==2,delete_tlblock(gcbh);end  NameChangeFcn=if exist('rename_tlblock','file')==2,rename_tlblock(gcbh);end  OpenFcn=if exist('tl_open_blockdlg','file')==2,tl_open_blockdlg(gcbh);else,open_system(gcbh,'parameter');end
      mask Help: eval(['if exist(''tl_online_help'',''file'') == 2, tl_online_help(''Topic'',''TL_RelationalOperator''),else, web([''jar:file:///'',matlabroot,''/help/toolbox/simulink/help.jar!/slref/' lower(get_param(gcbh,'Blocktype')) '.html''], ''-helpbrowser''),end'])
      mask Display: plot([-0.05, 1.05, NaN, -0.05, 1.05],[.01, .01, NaN, .99, .99])
  bInterruptStep : Outport  RequirementInfo={} %GIDa_90c1df2c_2ca8_4167_90df_05292780bb6b
  wires:
  s32BeltSpeed/1 -> RelationalOperator_bAccelerationLow/2
  B_TRUE/1 -> RelationalOperator_bAccelerationLow/1
  bBeltBlockedControlled/1 -> ManageBeltBlocked/1
  ManageBeltBlocked/1 -> bInterruptStep/1
  RelationalOperator_bAccelerationLow/1 -> ManageBeltBlocked/2

== system LIB_TF_G_12_StepControl/TF_G_12_ManageEndingStep/Step execution in progress/ManageBeltBlocked (HES sensors)/Belt Blocked Opt Deactivated ==
  Action Port : ActionPort  RequirementInfo={} %GIDa_8daab63d_3755_4e2f_849c_4036c52aad5c
  KB_FALSE : Constant  RequirementInfo={} %GIDa_1b7b36dc_bb90_4a92_bfa4_13cc0b838c4f  Value=ddv('BFE/KB_FALSE')  OutDataTypeStr=boolean  SampleTime=-1  mask(TL_Constant){data={'output',{'variable','BFE/KB_FALSE'},'date',735951.66847817134}}
      settings: CopyFcn=if exist('tl_reset_reviewflag','file')==2,tl_reset_reviewflag(gcbh);end  DeleteFcn=if exist('delete_tlblock','file')==2,delete_tlblock(gcbh);end  NameChangeFcn=if exist('rename_tlblock','file')==2,rename_tlblock(gcbh);end  OpenFcn=if exist('tl_open_blockdlg','file')==2,tl_open_blockdlg(gcbh);else,open_system(gcbh,'parameter');end
      mask Help: eval(['if exist(''tl_online_help'',''file'') == 2, tl_online_help(''Topic'',''TL_Constant''),else, web([''jar:file:///'',matlabroot,''/help/toolbox/simulink/help.jar!/slref/' lower(get_param(gcbh,'Blocktype')) '.html''], ''-helpbrowser''),end'])
      mask Display: plot([-0.05, 1.05, NaN, -0.05, 1.05],[.01, .01, NaN, .99, .99])
  bInterruptStep : Outport  RequirementInfo={} %GIDa_baca49a0_e277_4ce2_94d2_3ad032089136  InitialOutput=0
  wires:
  KB_FALSE/1 -> bInterruptStep/1

== system LIB_TF_G_12_StepControl/TF_G_12_ManageEndingStep/Step execution in progress/ManageBeltMvtDetection (HES sensors)/Belt Mvt Detect Opt Activated ==
  bBeltMvtDetection : Inport  RequirementInfo={} %GIDa_c0e90ffb_ae55_4ea1_aa14_4d9b7451ea0c
  s32BeltSpeed : Inport  RequirementInfo={} %GIDa_457d2d90_513a_46ff_ae64_0bf1c41735eb  Port=2
  Action Port : ActionPort  RequirementInfo={} %GIDa_0dae55cb_bf5a_4f27_9f1e_94df0ca7add1
  B_TRUE : Constant  RequirementInfo={} %GIDa_b8757e30_b53a_4d4d_b43e_62cbea956132  Value=ddv('Common/KS32_ZERO')  OutDataTypeStr=int32  SampleTime=-1  mask(TL_Constant){data={'output',{'variable','Common/KS32_ZERO'},'date',735951.66847692127}}
      settings: CopyFcn=if exist('tl_reset_reviewflag','file')==2,tl_reset_reviewflag(gcbh);end  DeleteFcn=if exist('delete_tlblock','file')==2,delete_tlblock(gcbh);end  NameChangeFcn=if exist('rename_tlblock','file')==2,rename_tlblock(gcbh);end  OpenFcn=if exist('tl_open_blockdlg','file')==2,tl_open_blockdlg(gcbh);else,open_system(gcbh,'parameter');end
      mask Help: eval(['if exist(''tl_online_help'',''file'') == 2, tl_online_help(''Topic'',''TL_Constant''),else, web([''jar:file:///'',matlabroot,''/help/toolbox/simulink/help.jar!/slref/' lower(get_param(gcbh,'Blocktype')) '.html''], ''-helpbrowser''),end'])
      mask Display: plot([-0.05, 1.05, NaN, -0.05, 1.05],[.01, .01, NaN, .99, .99])
  ManageBeltMvt : Logic  RequirementInfo={} %GIDa_d5984a09_8762_40c1_acd0_e5127868ec10  AllPortsSameDT=off  OutDataTypeStr=boolean  mask(TL_LogicalOperator){data={'date',735951.66847656248}}
      settings: DeleteFcn=if exist('delete_tlblock','file')==2,delete_tlblock(gcbh);end  NameChangeFcn=if exist('rename_tlblock','file')==2,rename_tlblock(gcbh);end  OpenFcn=if exist('tl_open_blockdlg','file')==2,tl_open_blockdlg(gcbh);else,open_system(gcbh,'parameter');end
      mask Help: eval(['if exist(''tl_online_help'',''file'') == 2, tl_online_help(''Topic'',''TL_LogicalOperator''),else, web([''jar:file:///'',matlabroot,''/help/toolbox/simulink/help.jar!/slref/' lower(get_param(gcbh,'Blocktype')) '.html''], ''-helpbrowser''),end'])
      mask Display: plot([-0.05, 1.05, NaN, -0.05, 1.05],[.01, .01, NaN, .99, .99])
  RelationalOperator_bAccelerationLow : RelationalOperator  RequirementInfo={} %GIDa_70ab118d_a367_4a56_be4b_56681cfd8b8c  Operator=~=  OutDataTypeStr=boolean  mask(TL_RelationalOperator){data={'date',735951.66847631941}}
      settings: DeleteFcn=if exist('delete_tlblock','file')==2,delete_tlblock(gcbh);end  NameChangeFcn=if exist('rename_tlblock','file')==2,rename_tlblock(gcbh);end  OpenFcn=if exist('tl_open_blockdlg','file')==2,tl_open_blockdlg(gcbh);else,open_system(gcbh,'parameter');end
      mask Help: eval(['if exist(''tl_online_help'',''file'') == 2, tl_online_help(''Topic'',''TL_RelationalOperator''),else, web([''jar:file:///'',matlabroot,''/help/toolbox/simulink/help.jar!/slref/' lower(get_param(gcbh,'Blocktype')) '.html''], ''-helpbrowser''),end'])
      mask Display: plot([-0.05, 1.05, NaN, -0.05, 1.05],[.01, .01, NaN, .99, .99])
  bInterruptStep : Outport  RequirementInfo={} %GIDa_3302bd4e_c1d0_45a2_acd6_0c99f305c0b5
  wires:
  RelationalOperator_bAccelerationLow/1 -> ManageBeltMvt/2
  ManageBeltMvt/1 -> bInterruptStep/1
  bBeltMvtDetection/1 -> ManageBeltMvt/1
  B_TRUE/1 -> RelationalOperator_bAccelerationLow/1
  s32BeltSpeed/1 -> RelationalOperator_bAccelerationLow/2

== system LIB_TF_G_12_StepControl/TF_G_12_ManageEndingStep/Step execution in progress/ManageBeltMvtDetection (HES sensors)/Belt Mvt Detect Opt Deactivated ==
  Action Port : ActionPort  RequirementInfo={} %GIDa_592965ef_5c5a_4e42_8649_4a3523d5a22f
  KB_FALSE : Constant  RequirementInfo={} %GIDa_5c4dad68_87e5_41ae_ae7b_bf387b915a11  Value=ddv('BFE/KB_FALSE')  OutDataTypeStr=boolean  SampleTime=-1  mask(TL_Constant){data={'output',{'variable','BFE/KB_FALSE'},'date',735951.66847604164}}
      settings: CopyFcn=if exist('tl_reset_reviewflag','file')==2,tl_reset_reviewflag(gcbh);end  DeleteFcn=if exist('delete_tlblock','file')==2,delete_tlblock(gcbh);end  NameChangeFcn=if exist('rename_tlblock','file')==2,rename_tlblock(gcbh);end  OpenFcn=if exist('tl_open_blockdlg','file')==2,tl_open_blockdlg(gcbh);else,open_system(gcbh,'parameter');end
      mask Help: eval(['if exist(''tl_online_help'',''file'') == 2, tl_online_help(''Topic'',''TL_Constant''),else, web([''jar:file:///'',matlabroot,''/help/toolbox/simulink/help.jar!/slref/' lower(get_param(gcbh,'Blocktype')) '.html''], ''-helpbrowser''),end'])
      mask Display: plot([-0.05, 1.05, NaN, -0.05, 1.05],[.01, .01, NaN, .99, .99])
  bInterruptStep : Outport  RequirementInfo={} %GIDa_17862e08_aa2d_418b_bf98_11d7bb4158bb  InitialOutput=0
  wires:
  KB_FALSE/1 -> bInterruptStep/1
